simulink model "DVA"  (R2016a)
settings: Solver=VariableStepAuto  StartTime=0.0  StopTime=10.0  RelTol=1e-3
values from neighbouring files (symbols this model uses):
  c = 500    [main.m]
  ca = 50    [main.m]
  k = 200000    [main.m]
  ka = 10000    [main.m]
  M = 200    [main.m]
  m = 10    [main.m]
settings Model: Creator=rohit  LastModifiedBy=rohit
settings DataIOCC: SaveFormat=Array

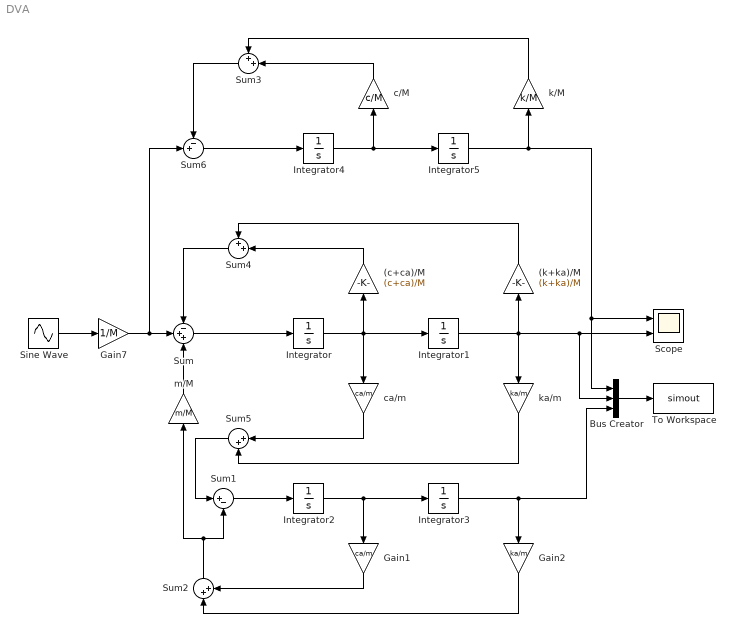
== system DVA ==
  (c+ca)/M : Gain  Gain=(c+ca)/M
  (k+ka)/M : Gain  Gain=(k+ka)/M
  Bus Creator : BusCreator  Inputs=3
  Gain1 : Gain  Gain=ca/m
  Gain2 : Gain  Gain=ka/m
  Gain7 : Gain  Gain=1/M
  Integrator{,1..5} (6 alike) : Integrator
  Scope : Scope  NumInputPorts=2
  Sine Wave : Sin  Amplitude=5000  Frequency=31.4  SampleTime=0
  Sum : Sum  Inputs=-++
  Sum1 : Sum  Inputs=|+-
  Sum2 : Sum  Inputs=|++
  Sum3 : Sum  Inputs=++|
  Sum4 : Sum  Inputs=++|
  Sum5 : Sum  Inputs=|++
  Sum6 : Sum  Inputs=-+|
  To Workspace : ToWorkspace  VariableName=simout  SaveFormat=Timeseries  SampleTime=-1
  c/M : Gain  Gain=c/M
  ca/m : Gain  Gain=ca/m
  k/M : Gain  Gain=k/M
  ka/m : Gain  Gain=ka/m
  m/M : Gain  Gain=m/M
  wires:
  Integrator/1 -> ca/m/1, Integrator1/1, (c+ca)/M/1
  Sum1/1 -> Integrator2/1
  Integrator2/1 -> Gain1/1, Integrator3/1
  Integrator3/1 -> Bus Creator/3, Gain2/1
  Gain1/1 -> Sum2/2
  Gain2/1 -> Sum2/1
  Integrator1/1 -> Bus Creator/2, Scope/2, (k+ka)/M/1, ka/m/1
  (k+ka)/M/1 -> Sum4/1
  (c+ca)/M/1 -> Sum4/2
  Sine Wave/1 -> Gain7/1
  Sum4/1 -> Sum/1
  ca/m/1 -> Sum5/1
  ka/m/1 -> Sum5/2
  Sum5/1 -> Sum1/1
  Sum/1 -> Integrator/1
  Gain7/1 -> Sum6/2, Sum/2
  Sum2/1 -> Sum1/2, m/M/1
  m/M/1 -> Sum/3
  Integrator4/1 -> Integrator5/1, c/M/1
  Integrator5/1 -> k/M/1, Bus Creator/1, Scope/1
  k/M/1 -> Sum3/1
  c/M/1 -> Sum3/2
  Sum6/1 -> Integrator4/1
  Sum3/1 -> Sum6/1
  Bus Creator/1 -> To Workspace/1
